simulink model "prog2"  (R2015b)
settings: Solver=ode45  StartTime=0.0  StopTime=0.1  FixedStep=0.0000001  RelTol=1e-9  AbsTol=1e-9
libraries: simulink x1
settings Model: Creator=zap  LastModifiedBy=zap

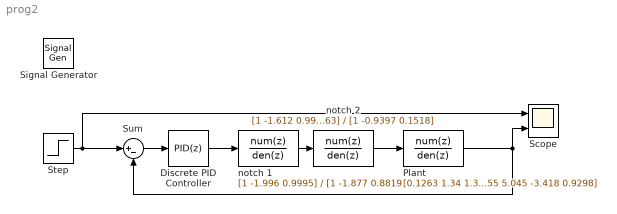
== system prog2 ==
  Discrete PID Controller : simulink/Continuous/PID Controller  Controller=PID  TimeDomain=Discrete-time  SampleTime=10^-4  IntegratorMethod=Forward Euler  FilterMethod=Forward Euler  Form=Parallel  UseFilter=on  ControllerParametersSource=internal  P=0.0015  I=0.2  D=0  N=100  InitialConditionSource=internal  InitialConditionForIntegrator=0  InitialConditionForFilter=0  ExternalReset=none  LimitOutput=off  UpperSaturationLimit=inf  LowerSaturationLimit=-inf  LinearizeAsGain=off  AntiWindupMode=none  Kb=1  TrackingMode=off  Kt=1  PParamMin=[]  PParamMax=[]  IParamMin=[]  IParamMax=[]  DParamMin=[]  DParamMax=[]  NParamMin=[]  NParamMax=[]  KbParamMin=[]  KbParamMax=[]  KtParamMin=[]  KtParamMax=[]  POutMin=[]  POutMax=[]  IOutMin=[]  IOutMax=[]  DOutMin=[]  DOutMax=[]  NOutMin=[]  NOutMax=[]  KbOutMin=[]  KbOutMax=[]  KtOutMin=[]  KtOutMax=[]  IntegratorOutMin=[]  IntegratorOutMax=[]  FilterOutMin=[]  FilterOutMax=[]  SumOutMin=[]  SumOutMax=[]  SumI1OutMin=[]  SumI1OutMax=[]  SumI2OutMin=[]  SumI2OutMax=[]  SumI3OutMin=[]  SumI3OutMax=[]  SumDOutMin=[]  SumDOutMax=[]  SaturationOutMin=[]  SaturationOutMax=[]  IntegratorContinuousStateAttributes=''  IntegratorStateMustResolveToSignalObject=off  IntegratorRTWStateStorageClass=Auto  FilterContinuousStateAttributes=''  FilterStateMustResolveToSignalObject=off  FilterRTWStateStorageClass=Auto  DifferentiatorICPrevScaledInput=0  DifferentiatorOutMin=[]  DifferentiatorOutMax=[]
  Plant : DiscreteTransferFcn  Numerator=[0.1263 1.34 1.32 0.1209]  Denominator=[1 -3.555 5.045 -3.418 0.9298]  SampleTime=10^-4
  Scope : Scope  NumInputPorts=2
  Signal Generator : SignalGenerator  WaveForm=square  Frequency=3  Units=rad/sec
  Step : Step  Time=0  SampleTime=10^-4
  Sum : Sum  Inputs=|+-
  notch 1 : DiscreteTransferFcn  Numerator=[1 -1.996 0.9995]  Denominator=[1 -1.877 0.8819]  SampleTime=10^-4
  notch 2 : DiscreteTransferFcn  Numerator=[1 -1.612 0.9963]  Denominator=[1 -0.9397 0.1518]  SampleTime=10^-4
  wires:
  Plant/1 -> Scope/2, Sum/2
  Sum/1 -> Discrete PID Controller/1
  Discrete PID Controller/1 -> notch 1/1
  notch 1/1 -> notch 2/1
  notch 2/1 -> Plant/1
  Step/1 -> Scope/1, Sum/1
